simulink model "Task_8_1"  (R2015a)
settings: Solver=ode45  StartTime=0.0  StopTime=10.0  RelTol=1e-3
settings Model: Creator=acer  LastModifiedBy=acer

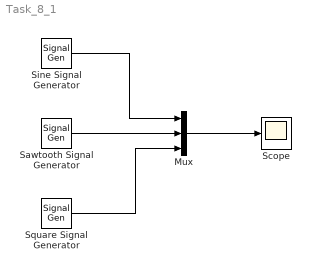
== system Task_8_1 ==
  Mux : Mux  Inputs=3
  Sawtooth Signal Generator : SignalGenerator  WaveForm=sawtooth  Units=rad/sec
  Scope : Scope
  Sine Signal Generator : SignalGenerator  Units=rad/sec
  Square Signal Generator : SignalGenerator  WaveForm=square  Units=rad/sec
  wires:
  Sawtooth Signal Generator/1 -> Mux/2
  Mux/1 -> Scope/1
  Sine Signal Generator/1 -> Mux/1
  Square Signal Generator/1 -> Mux/3
